simulink model "si3b_coilAC"  (R2024a)
settings: Solver=VariableStepAuto  StartTime=0.0  StopTime=te  MaxStep=te/500  RelTol=1e-3
values from neighbouring files (symbols this model uses):
  L = 1    [sim21_solution.m]
  R = 10    [sim21_solution.m]
  U = 230*sqrt(2)    [sim21_solution.m]
  w = [0.5 1 2]    [sim21_solution.m]
settings Model: Creator=ocean  LastModifiedBy=ocean

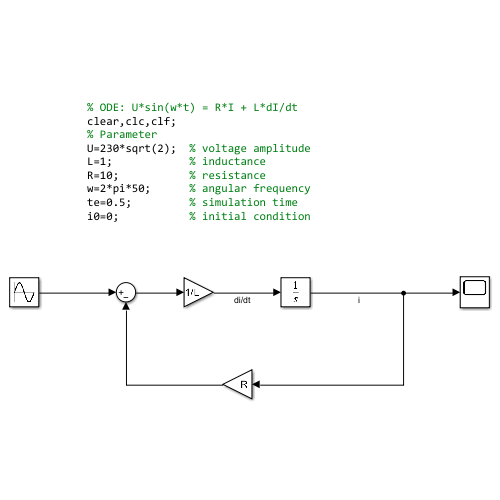
[thumbnail: Simulink's stored preview of the top-level diagram]
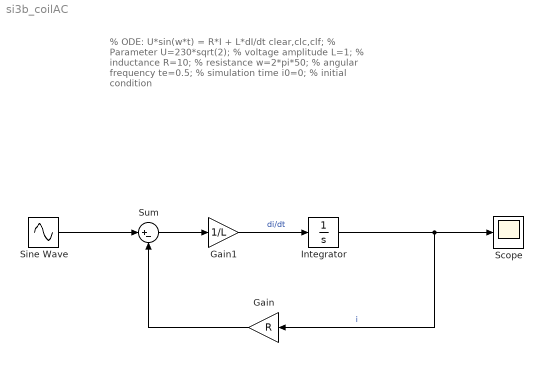
== system si3b_coilAC ==
  note: % ODE: U*sin(w*t) = R*I + L*dI/dt
      | clear,clc,clf;
      | % Parameter
      | U=230*sqrt(2); % voltage amplitude
      | L=1; % inductance
      | R=10; % resistance
      | w=2*pi*50; % angular frequency
      | te=0.5; % simulation time
      | i0=0; % initial condition
  Gain : Gain  Gain=R
  Gain1 : Gain  Gain=1/L
  Integrator : Integrator
  Scope : Scope
  Sine Wave : Sin  Amplitude=U  Frequency=w  SampleTime=0
  Sum : Sum  Inputs=|+-
  wires:
  Integrator/1 -> Gain/1, Scope/1  "i"
  Sine Wave/1 -> Sum/1
  Sum/1 -> Gain1/1
  Gain1/1 -> Integrator/1  "di/dt"
  Gain/1 -> Sum/2
